simulink model "IMUconversion"  (R2022b)
settings: Solver=VariableStepAuto  StartTime=0.0  StopTime=15.0  RelTol=1e-3
settings Model: Creator=husey  LastModifiedBy=husey

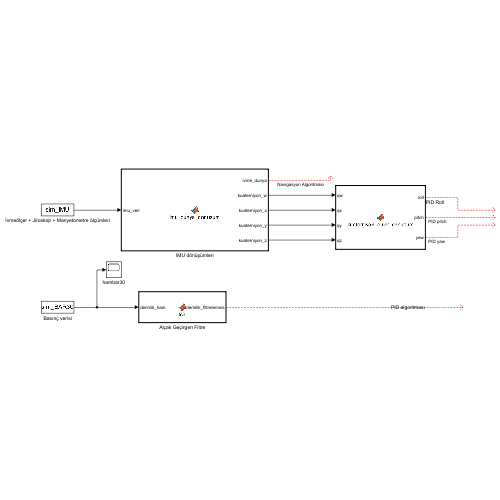
[thumbnail: Simulink's stored preview of the top-level diagram]
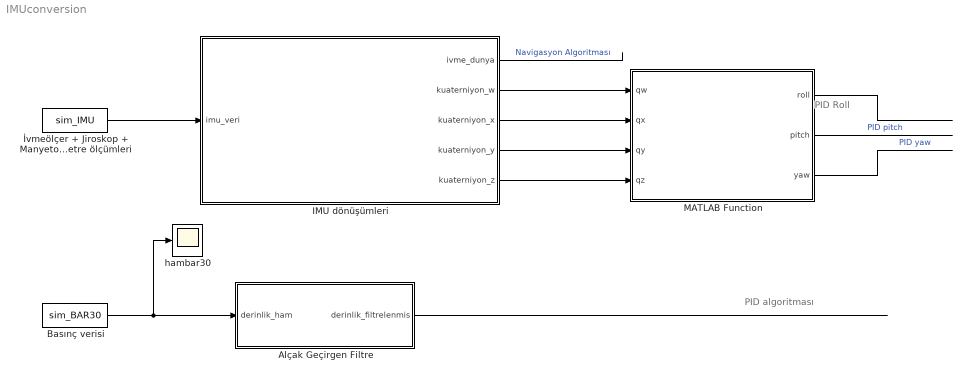
== system IMUconversion ==
  note: PID algoritması
  note: PID Roll
  Alçak Geçirgen Filtre : MATLAB Function  TreatAsAtomicUnit=on
  Basınç verisi : FromWorkspace  VariableName=sim_BAR30
  IMU dönüşümleri : MATLAB Function  TreatAsAtomicUnit=on
  MATLAB Function : MATLAB Function  TreatAsAtomicUnit=on
  hambar30 : Scope
  İvmeölçer + Jiroskop + Manyetometre ölçümleri : FromWorkspace  VariableName=sim_IMU
  wires:
  İvmeölçer + Jiroskop + Manyetometre ölçümleri/1 -> IMU dönüşümleri/1(imu_veri)
  IMU dönüşümleri/1(ivme_dunya) -> ?  "Navigasyon Algoritması"
  IMU dönüşümleri/2(kuaterniyon_w) -> MATLAB Function/1(qw)
  IMU dönüşümleri/5(kuaterniyon_z) -> MATLAB Function/4(qz)
  IMU dönüşümleri/4(kuaterniyon_y) -> MATLAB Function/3(qy)
  IMU dönüşümleri/3(kuaterniyon_x) -> MATLAB Function/2(qx)
  MATLAB Function/1(roll) -> ?
  MATLAB Function/2(pitch) -> ?  "PID pitch"
  MATLAB Function/3(yaw) -> ?  "PID yaw"
  Alçak Geçirgen Filtre/1(derinlik_filtrelenmis) -> ?
  Basınç verisi/1 -> hambar30/1, Alçak Geçirgen Filtre/1(derinlik_ham)

== matlab function IMUconversion/MATLAB Function ==
  data: qw input; roll output; qx input; qy input; qz input; pitch output; yaw output
function [roll, pitch, yaw] = kuaterniyon_euler_donusum(qw, qx, qy, qz)
    % Kuaterniyon (w, x, y, z) verisini Euler açılarına (Roll, Pitch, Yaw) dönüştürür.
    % Çıkışlar görselleştirme ve kontrol kolaylığı için DERECE cinsindendir.

    % 1. Roll (Yalpalama - X ekseni etrafında dönüş)
    sinr_cosp = 2 * (qw * qx + qy * qz);
    cosr_cosp = 1 - 2 * (qx^2 + qy^2);
    roll_rad = atan2(sinr_cosp, cosr_cosp);
    roll = roll_rad * (180.0 / pi);

    % 2. Pitch (Yunuslama - Y ekseni etrafında dönüş)
    sinp = 2 * (qw * qy - qz * qx);
    % Float hassasiyetinden kaynaklanabilecek NaN (Not a Number) hatalarını 
    % ve Gimbal Lock durumunu önlemek için sınırlandırma (clamping)
    if abs(sinp) >= 1
        pitch_rad = sign(sinp) * (pi / 2);
    else
        pitch_rad = asin(sinp);
    end
    pitch = pitch_rad * (180.0 / pi);

    % 3. Yaw (Sapma - Z ekseni etrafında dönüş)
    siny_cosp = 2 * (qw * qz + qx * qy);
    cosy_cosp = 1 - 2 * (qy^2 + qz^2);
    yaw_rad = atan2(siny_cosp, cosy_cosp);
    yaw = yaw_rad * (180.0 / pi);
end

== matlab function IMUconversion/IMU dönüşümleri ==
  data: imu_veri input; ivme_dunya output; kuaterniyon_w output; kuaterniyon_x output; kuaterniyon_y output; kuaterniyon_z output
function [ivme_dunya, kuaterniyon_w, kuaterniyon_x, kuaterniyon_y, kuaterniyon_z] = imu_dunya_donusum(imu_veri)
    % Giriş (Tek Port):
    %   imu_veri : 9 elemanlı float vektörü -> [ax; ay; az; gx; gy; gz; mx; my; mz]
    %
    % Çıkışlar:
    %   ivme_dunya       : Yerçekimi düşülmüş dünya ekseni ivmesi [X; Y; Z] (m/s^2)
    %   kuaterniyon_w, kuaterniyon_x, kuaterniyon_y, kuaterniyon_z : Yönelim kuaterniyonunun bağımsız bileşenleri

    % Sistem zaman adımı (200 Hz için sabit)
    dt = 0.005;

    % 1. Tekil giriş vektöründen (9 float) verilerin ayrıştırılması
    ivme_ham         = imu_veri(1:3);
    jiroskop_ham     = imu_veri(4:6);
    manyetometre_ham = imu_veri(7:9);

    % 2. Kalıcı (Persistent) Değişken Tanımı
    persistent q baslatildi
    if isempty(baslatildi)
        q = [1; 0; 0; 0]; % Başlangıç kuaterniyonu [w; x; y; z]
        baslatildi = true;
    end

    % 3. Giriş Verilerinin Normalizasyonu (Sıfıra bölünme korumalı)
    norm_a = sqrt(ivme_ham(1)^2 + ivme_ham(2)^2 + ivme_ham(3)^2);
    if norm_a == 0, norm_a = 1; end
    ax = ivme_ham(1)/norm_a; ay = ivme_ham(2)/norm_a; az = ivme_ham(3)/norm_a;

    norm_m = sqrt(manyetometre_ham(1)^2 + manyetometre_ham(2)^2 + manyetometre_ham(3)^2);
    if norm_m == 0, norm_m = 1; end
    mx = manyetometre_ham(1)/norm_m; my = manyetometre_ham(2)/norm_m; mz = manyetometre_ham(3)/norm_m;

    q0 = q(1); q1 = q(2); q2 = q(3); q3 = q(4);

    % 4. Jiroskop Verisi ile Yönelim İntegrasyonu 
    q_nokta = 0.5 * [ -q1*jiroskop_ham(1) - q2*jiroskop_ham(2) - q3*jiroskop_ham(3);
                       q0*jiroskop_ham(1) - q3*jiroskop_ham(2) + q2*jiroskop_ham(3);
                       q3*jiroskop_ham(1) + q0*jiroskop_ham(2) - q1*jiroskop_ham(3);
                      -q2*jiroskop_ham(1) + q1*jiroskop_ham(2) + q0*jiroskop_ham(3) ];

    % 5. Manyetometre Düzeltmesi ve Referans Alan Hesabı
    hx = mx*(q0^2 + q1^2 - q2^2 - q3^2) + 2*my*(q1*q2 - q0*q3) + 2*mz*(q1*q3 + q0*q2);
    hy = 2*mx*(q1*q2 + q0*q3) + my*(q0^2 - q1^2 + q2^2 - q3^2) + 2*mz*(q2*q3 - q0*q1);
    bx = sqrt(hx^2 + hy^2);
    bz = 2*mx*(q1*q3 - q0*q2) + 2*my*(q2*q3 + q0*q1) + mz*(q0^2 - q1^2 - q2^2 + q3^2);

    % Hata Fonksiyonu
    f = [ 2*(q1*q3 - q0*q2) - ax;
          2*(q0*q1 + q2*q3) - ay;
          2*(0.5 - q1^2 - q2^2) - az;
          2*bx*(0.5 - q2^2 - q3^2) + 2*bz*(q1*q3 - q0*q2) - mx;
          2*bx*(q1*q2 - q0*q3) + 2*bz*(q0*q1 + q2*q3) - my;
          2*bx*(q0*q2 + q1*q3) + 2*bz*(0.5 - q1^2 - q2^2) - mz ];

    % Jacobian Matrisi
    J = [ -2*q2,  2*q3, -2*q0,  2*q1;
           2*q1,  2*q0,  2*q3,  2*q2;
           0,    -4*q1, -4*q2,  0;
          -2*bz*q2, 2*bz*q3, -4*bx*q2-2*bz*q0, -4*bx*q3+2*bz*q1;
          -2*bx*q3+2*bz*q1, 2*bx*q2+2*bz*q0, 2*bx*q1+2*bz*q3, -2*bx*q0+2*bz*q2;
           2*bx*q2-4*bz*q1, 2*bx*q3-4*bz*q2, 2*bx*q0,  2*bx*q1 ];

    adim = J' * f;
    norm_adim = sqrt(adim(1)^2 + adim(2)^2 + adim(3)^2 + adim(4)^2);
    if norm_adim > 0
        adim = adim / norm_adim;
    end

    % 6. Kuaterniyon Güncelleme ve Normalizasyon
    beta = 0.1; % Filtre kazancı
    q_nokta = q_nokta - beta * adim;
    
    q = q + q_nokta * dt;
    q = q / sqrt(q(1)^2 + q(2)^2 + q(3)^2 + q(4)^2);

    % --- ÇIKIŞ 1: KUATERNİYON BİLEŞENLERİNİN AYRILMASI ---
    kuaterniyon_w = q(1);
    kuaterniyon_x = q(2);
    kuaterniyon_y = q(3);
    kuaterniyon_z = q(4);

    % --- ÇIKIŞ 2: DÜNYA EKSENİNE DÖNÜŞÜM ---
    % Gövde ekseninden dünya eksenine dönüşüm matrisi (R)
    R = [ kuaterniyon_w^2+kuaterniyon_x^2-kuaterniyon_y^2-kuaterniyon_z^2,   2*(kuaterniyon_x*kuaterniyon_y-kuaterniyon_w*kuaterniyon_z),       2*(kuaterniyon_x*kuaterniyon_z+kuaterniyon_w*kuaterniyon_y);
          2*(kuaterniyon_x*kuaterniyon_y+kuaterniyon_w*kuaterniyon_z),       kuaterniyon_w^2-kuaterniyon_x^2+kuaterniyon_y^2-kuaterniyon_z^2,   2*(kuaterniyon_y*kuaterniyon_z-kuaterniyon_w*kuaterniyon_x);
          2*(kuaterniyon_x*kuaterniyon_z-kuaterniyon_w*kuaterniyon_y),       2*(kuaterniyon_y*kuaterniyon_z+kuaterniyon_w*kuaterniyon_x),       kuaterniyon_w^2-kuaterniyon_x^2-kuaterniyon_y^2+kuaterniyon_z^2 ];

    % Yerçekimini temizle ve saf lineer ivmeyi bul
    ivme_dunya_ham = R * ivme_ham(:); 
    ivme_dunya = ivme_dunya_ham - [0; 0; 9.81];
end

== matlab function IMUconversion/Alçak Geçirgen Filtre ==
  data: derinlik_ham input; derinlik_filtrelenmis output
function derinlik_filtrelenmis = fcn(derinlik_ham)
    % #--- BAR30 İÇİN ALÇAK GEÇİREN FİLTRE (LOW-PASS FILTER) ---#
    % Giriş:
    %   derinlik_ham : Sensörden gelen gürültülü anlık ölçüm
    % Çıkış:
    %   derinlik_filtrelenmis : Gürültüden arındırılmış pürüzsüz derinlik

    % 1. Filtre Katsayısı (Alpha: 0 ile 1 arasında)
    % Alpha = 1  -> Hiç filtreleme yapmaz, ham veriyi doğrudan geçirir.
    % Alpha = 0  -> Tamamen dondurur, veri hiç değişmez.
    % Tavsiye: 200 Hz (dt=0.005) çalışan bir derinlik sensörü için 0.05 ile 0.1 arası idealdir.
    alpha = 0.05; 

    % 2. Hafıza (Geçmiş değerin tutulması)
    persistent derinlik_eski baslatildi

    % Sistem ilk çalıştığında filtrenin sıfırdan hedefe fırlamasını (sıçrama) 
    % önlemek için ilk değeri doğrudan ham veriye eşitliyoruz.
    if isempty(baslatildi)
        derinlik_eski = derinlik_ham; 
        baslatildi = true;
    end

    % 3. Alçak Geçiren Filtre Denklemi
    derinlik_filtrelenmis = alpha * derinlik_ham + (1 - alpha) * derinlik_eski;

    % 4. Bir Sonraki Adım İçin Hafızayı Güncelle
    derinlik_eski = derinlik_filtrelenmis;
end
